simulink model "MotorPD_simonly_Student"  (R2025a)
settings: Solver=FixedStepAuto  StartTime=0.0  StopTime=20  FixedStep=0.002  RelTol=1e-3  EnableMultiTasking=on
undefined symbols (not defined in the file): K, tau
settings Model: ExtModeTrigDuration=10000  Creator=LabRyu  LastModifiedBy=User
settings SolverCC: AlgebraicLoopSolver=TrustRegion  PositivePriorityOrder=on
settings DataIOCC: ReturnWorkspaceOutputs=off
settings DebuggingCC: UnconnectedInputMsg=warning  UnconnectedOutputMsg=warning  UnconnectedLineMsg=warning  ArithmeticOperatorsInVariantConditions=warning
settings ModelReferenceCC: EnableRefExpFcnMdlSchedulingChecks=on
settings SFSimCC: SimUseLocalCustomCode=off  CustomCodeUndefinedFunction=UseInterfaceOnly
settings RTWCC: SystemTargetFile=quarc_win64.tlc  TemplateMakefile=quarc_default_tmf  RTWUseLocalCustomCode=off  GPUComputeCapability=3.5  Description=QUARC Win64 Target
settings CodeAppCC: StateflowObjectComments=on
settings STFCustomTargetCC: SystemTargetFile=quarc_win64.tlc  TargetPreCompLibLocation=C:\PROGRA~3\QUARC\lib\2017a\win64\release  TargetLangStandard=C99 (ISO)  MultiwordLength=2048.0  DynamicStringBufferSize=256.0  ConcurrentExecutionCompliant=on  DownloadToTarget=on  StopOnOverrun=off  Debug=off
settings GRTTargetCC: ExtMode=on  ExtModeMexFile=quarc_comm  TargetPreCompLibLocation=C:\PROGRA~3\QUARC\lib\2017a\win64\release  ParMdlRefBuildCompliant=off  CompOptLevelCompliant=off  CombineOutputUpdateFcns=off  MatFileLogging=off  CPPClassGenCompliant=off  GRTInterface=on  UseToolchainInfoCompliant=off

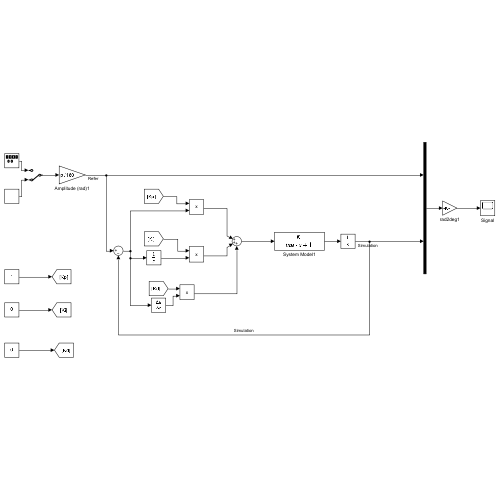
[thumbnail: Simulink's stored preview of the top-level diagram]
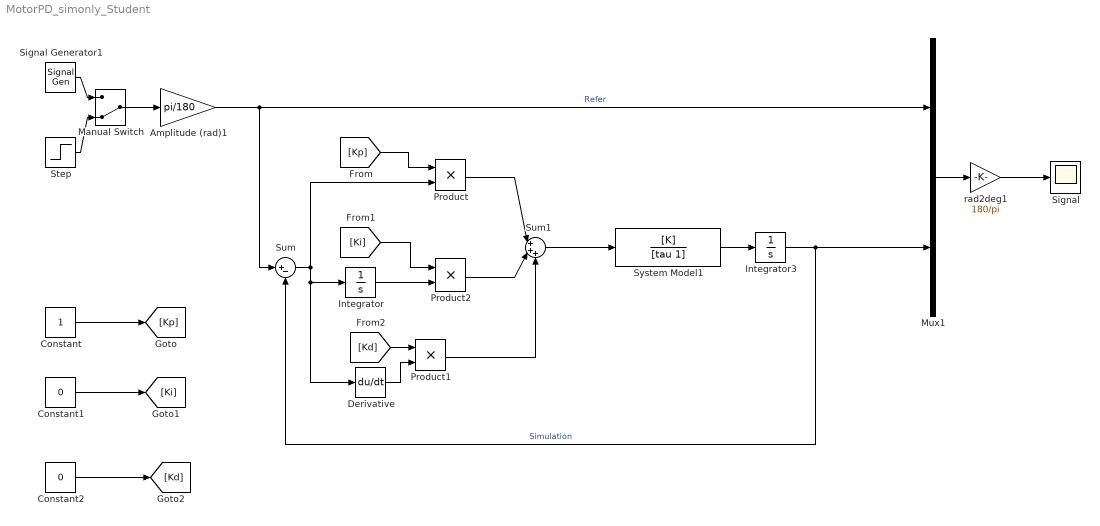
== system MotorPD_simonly_Student ==
  Amplitude (rad)1 : Gain  Gain=pi/180
  Constant : Constant
  Constant1 : Constant  Value=0
  Constant2 : Constant  Value=0
  Derivative : Derivative
  Integrator : Integrator
  Integrator3 : Integrator
  Manual Switch : ManualSwitch  CurrentSetting=0
  Mux1 : Mux  Inputs=2
  Product : Product
  Product1 : Product
  Product2 : Product
  Signal : Scope
      settings: TimeSpan=20  ActiveDisplayYMinimum=-1.4604111262699284  ActiveDisplayYMaximum=2.7096128658814758  DataLoggingMaxPoints=25000  DataLoggingSaveFormat=Array
  Signal Generator1 : SignalGenerator  WaveForm=square  Amplitude=45  Frequency=0.1
  Step : Step  SampleTime=0
  Sum : Sum  Inputs=|+-
  Sum1 : Sum  Inputs=|+++
  System Model1 : TransferFcn  Numerator=[K]  Denominator=[tau 1]
  rad2deg1 : Gain  Gain=180/pi
  wires:
  Mux1/1 -> rad2deg1/1
  rad2deg1/1 -> Signal/1
  Amplitude (rad)1/1 -> Sum/1, Mux1/1  "Refer"
  System Model1/1 -> Integrator3/1
  Integrator3/1 -> Mux1/2, Sum/2  "Simulation"
  Signal Generator1/1 -> Manual Switch/1
  Step/1 -> Manual Switch/2
  Manual Switch/1 -> Amplitude (rad)1/1
  Constant/1 -> [Kp]
  Constant1/1 -> [Ki]
  Constant2/1 -> [Kd]
  [Kp] -> Product/1
  Derivative/1 -> Product1/2
  Sum/1 -> Product/2, Derivative/1, Integrator/1
  [Kd] -> Product1/1
  [Ki] -> Product2/1
  Sum1/1 -> System Model1/1
  Product/1 -> Sum1/1
  Integrator/1 -> Product2/2
  Product1/1 -> Sum1/3
  Product2/1 -> Sum1/2
